simulink model "Ex31"  (R2021b)
settings: Solver=VariableStepAuto  StartTime=0.0  StopTime=10.0  RelTol=1e-3
settings Model: Creator=abdul  LastModifiedBy=abdul

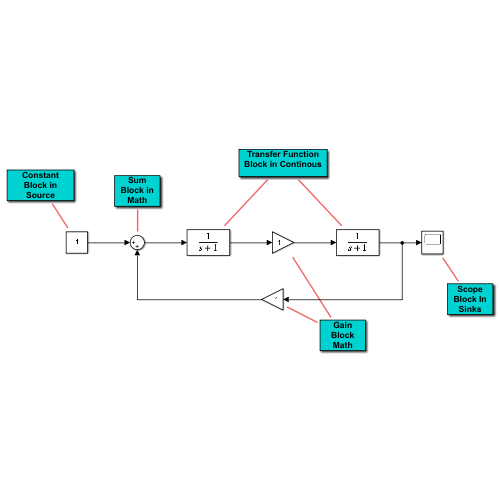
[thumbnail: Simulink's stored preview of the top-level diagram]
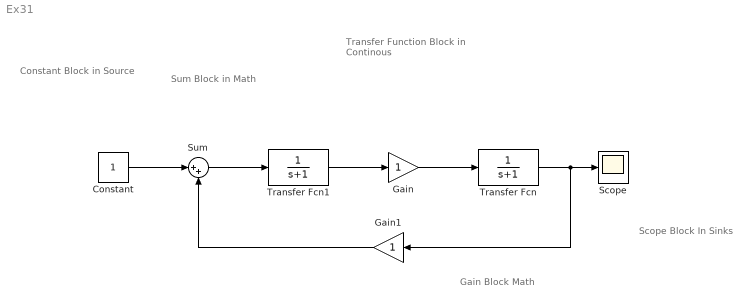
== system Ex31 ==
  note: Constant Block in Source
  note: Sum Block in Math
  note: Transfer Function Block in Continous
  note: Gain Block Math
  note: Scope Block In Sinks
  Constant : Constant
  Gain : Gain
  Gain1 : Gain
  Scope : Scope
  Sum : Sum  Inputs=|++
  Transfer Fcn : TransferFcn  Denominator=[1 1]
  Transfer Fcn1 : TransferFcn  Denominator=[1 1]
  wires:
  Sum/1 -> Transfer Fcn1/1
  Transfer Fcn1/1 -> Gain/1
  Gain/1 -> Transfer Fcn/1
  Gain1/1 -> Sum/2
  Transfer Fcn/1 -> Gain1/1, Scope/1
  Constant/1 -> Sum/1
